simulink model "mcb_pmsm_foc_dual_host_model"  (R2024b)
settings: Solver=FixedStepDiscrete  StartTime=0.0  StopTime=inf  RelTol=1e-3  EnableMultiTasking=on
values from neighbouring files (symbols this model uses):
  dataType = 'single'    [mcb_pmsm_foc_dual_f28379d_datascript.m]    (also in mcb_pmsm_foc_sensorless_dyno_f28379d_datascript.m)
  PU_System = mcb_SetPUSystem(pmsm,inverter)    [mcb_pmsm_foc_dual_f28379d_datascript.m]
  Ts = T_pwm    (= 5e-05)    [mcb_pmsm_foc_dual_f28379d_datascript.m]    (also in mcb_pmsm_foc_sensorless_dyno_f28379d_datascript.m)
libraries: instrumentseriallib x4, simulink x3, demo_controls x1
settings Model: Creator=The MathWorks, Inc.  LastModifiedBy=36961
settings SolverCC: AlgebraicLoopSolver=TrustRegion  MaxZcPerStep=1
settings DataIOCC: LimitDataPoints=on  SaveFormat=Array  ReturnWorkspaceOutputs=off
settings OptimizationCC: LifeSpan=1  EfficientTunableParamExpr=on
settings DebuggingCC: UnderspecifiedInitializationDetection=Classic  MergeDetectMultiDrivingBlocksExec=none  SolverPrmCheckMsg=warning  ParameterPrecisionLossMsg=none  UnconnectedInputMsg=warning  UnconnectedOutputMsg=warning  UnconnectedLineMsg=warning  AllowSymbolicDim=off  PregeneratedLibrarySubsystemCodeDiagnostic=none  SFUnexpectedBacktrackingDiag=warning  SFNoUnconditionalDefaultTransitionDiag=warning  SFExecutionAtInitializationDiag=none  ArithmeticOperatorsInVariantConditions=warning
settings HardwareCC: ProdBitPerPointer=32  ProdLargestAtomicFloat=None  ProdIntDivRoundTo=Undefined  ProdEndianess=Unspecified  ProdWordSize=32  ProdHWDeviceType=32-bit Generic
settings ModelReferenceCC: EnableRefExpFcnMdlSchedulingChecks=on  PropagateSignalLabelsOutOfModel=off
settings SFSimCC: SimUseLocalCustomCode=off  MATLABDynamicMemAlloc=off
settings RTWCC: Description=Real-Time Workshop Embedded Coder  SystemTargetFile=ert.tlc  TemplateMakefile=ert_default_tmf  GenerateReport=on  RTWUseLocalCustomCode=off  IncludeHyperlinkInReport=on  LaunchReport=on  GenerateTraceInfo=on  GenerateTraceReport=on  GenerateTraceReportSl=on  GenerateTraceReportSf=on  GenerateTraceReportEml=on  GPUComputeCapability=3.5  DLArmComputeVersion=19.05
settings CodeAppCC: IgnoreCustomStorageClasses=off  StateflowObjectComments=on  InternalIdentifier=Classic
settings ERTTargetCC: MultiwordLength=2048  GenerateSampleERTMain=on  InlinedParameterPlacement=Hierarchical  ERTCustomFileTemplate=example_file_process.tlc  ConvertIfToSwitch=off  SuppressUnreachableDefaultCases=off  DynamicArrayContainerType=coder::array
settings ConfigComp: CovMetricSettings=dw  CovSaveCumulativeToWorkspaceVar=on  CovSaveSingleToWorkspaceVar=on  CovExternalEMLEnable=off  CovSFcnEnable=off

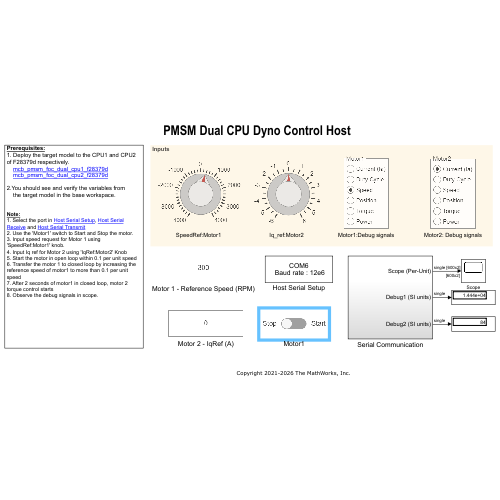
[thumbnail: Simulink's stored preview of the top-level diagram]
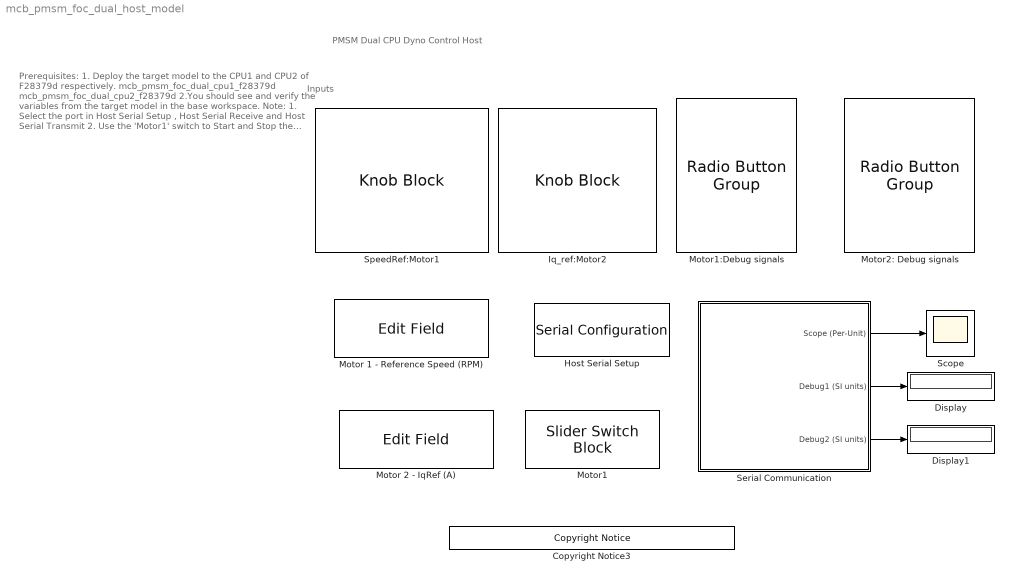
== system mcb_pmsm_foc_dual_host_model ==
  note: PMSM Dual CPU Dyno Control Host
  note: Prerequisites:
      | 1. Deploy the target model to the CPU1 and CPU2 of F28379d respectively.
      | mcb_pmsm_foc_dual_cpu1_f28379d
      | mcb_pmsm_foc_dual_cpu2_f28379d
      |
      | 2.You should see and verify the variables from
      | the target model in the base workspace.
      |
      | Note:
      | 1. Select the port in Host Serial Setup , Host Serial Receive and Host Serial Transmit
      | 2. Use the 'Motor1' switch to Start and Stop the motor.
      | 3. Input speed request for Motor 1 using 'SpeedRef:Motor1' knob.
      | 4. Input Iq ref for Motor 2 using 'IqRef:Motor2' Knob
      | 5. Start the motor in open loop within 0.1 per unit speed
      | 6. Transfer the motor 1 to closed loop by increasing the reference speed of motor1 to more than 0.1 per unit speed
      | 7. After 2 seconds of motor1 in closed loop, motor 2 torque control starts
      | 8. Observe the debug signals in scope.
  note: Inputs
  Copyright Notice3 : demo_controls/Copyright Notice  year=2021  prod=tic2000
  Display : Display
  Display1 : Display
  Host Serial Setup : instrumentseriallib/Serial Configuration  Priority=-99  PortSel=COM6  Port=COM6  ComPort=COM6  BaudRate=12e6  DataBits=8  Parity=none  StopBits=1  ByteOrder=little-endian  FlowControl=none  Timeout=2  SimulateUsing=Interpreted execution  BlockInModel=on  aMode=5
  Iq_ref:Motor2 : KnobBlock  LabelPosition=Hide  ScaleMin=-6  ScaleMax=6
  Motor 1 - Reference Speed (RPM) : EditField  LabelPosition=Hide  ShowInitialText=on  Alignment=Center
  Motor 2 - IqRef (A) : EditField  LabelPosition=Hide  ShowInitialText=on  Alignment=Center
  Motor1 : SliderSwitchBlock  LabelPosition=Hide
      settings: Values={{'Stop', 'Start'}, [0 1]}
  Motor1:Debug signals : RadioButtonGroup  LabelPosition=Hide  SelectedLabel=Speed  ButtonGroupName=Motor1
      settings: Values={{'Current (Ia)', 'Duty Cycle', 'Speed', 'Position', 'Torque', 'Power'}, [0 1 2 3 4 5]}
  Motor2: Debug signals : RadioButtonGroup  LabelPosition=Hide  SelectedLabel=Current (Ia)  ButtonGroupName=Motor2
      settings: Values={{'Current (Ia)', 'Duty Cycle', 'Speed', 'Position', 'Torque', 'Power'}, [0 1 2 3 4 5]}
  Scope : Scope
  Serial Communication : Subsystem
  SpeedRef:Motor1 : KnobBlock  LabelPosition=Hide  ScaleMin=-4000  ScaleMax=4000
  wires:
  Serial Communication/2(Debug1 (SI units)) -> Display/1
  Serial Communication/3(Debug2 (SI units)) -> Display1/1
  Serial Communication/1(Scope (Per-Unit)) -> Scope/1

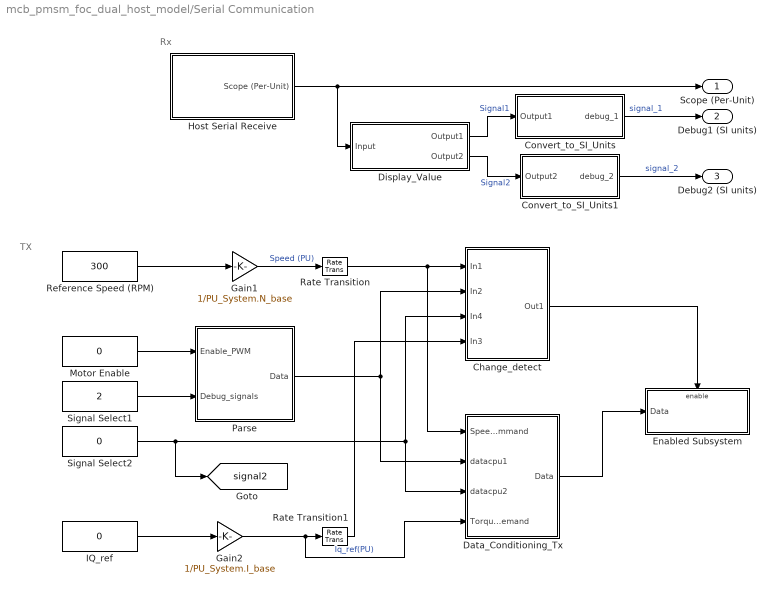
== system mcb_pmsm_foc_dual_host_model/Serial Communication ==
  note: TX
  note: Rx
  Change_detect : Subsystem
  Convert_to_SI_Units : Subsystem
  Convert_to_SI_Units1 : Subsystem
  Data_Conditioning_Tx : Subsystem  Variant=on
  Display_Value : MATLAB Function  TreatAsAtomicUnit=on
  Enabled Subsystem : Subsystem  TreatAsAtomicUnit=on
  Gain1 : Gain  Gain=1/PU_System.N_base  RndMeth=Simplest  OutDataTypeStr=Inherit: Same as input
  Gain2 : Gain  Gain=1/PU_System.I_base  RndMeth=Simplest  OutDataTypeStr=Inherit: Same as input
  Host Serial Receive : Subsystem  Variant=on
  IQ_ref : Constant  Value=0  VectorParams1D=off  OutDataTypeStr=single  SampleTime=0.03
  Motor Enable : Constant  Value=0  VectorParams1D=off  OutDataTypeStr=uint16  SampleTime=0.03
  Parse : Subsystem
  Rate Transition : RateTransition  OutPortSampleTime=0.03
  Rate Transition1 : RateTransition  OutPortSampleTime=0.03
  Reference Speed (RPM) : Constant  Value=300  VectorParams1D=off  OutDataTypeStr=single  SampleTime=0.03
  Signal Select1 : Constant  Value=2  OutDataTypeStr=uint16  SampleTime=0.03
  Signal Select2 : Constant  Value=0  OutDataTypeStr=uint16  SampleTime=0.03
  Scope (Per-Unit) : Outport
  Debug1 (SI units) : Outport  Port=2
  Debug2 (SI units) : Outport  Port=3
  tag scope: signal2=global
  wires:
  Reference Speed (RPM)/1 -> Gain1/1
  Gain2/1 -> Data_Conditioning_Tx/4(TorqueDemand), Rate Transition1/1  "Iq_ref(PU)"
  Parse/1(Data) -> Change_detect/2(In2), Data_Conditioning_Tx/2(datacpu1)
  Change_detect/1(Out1) -> Enabled Subsystem/Enable
  Data_Conditioning_Tx/1(Data) -> Enabled Subsystem/1(Data)
  Signal Select2/1 -> [signal2], Data_Conditioning_Tx/3(datacpu2), Change_detect/3(In4)
  Rate Transition1/1 -> Change_detect/4(In3)
  Motor Enable/1 -> Parse/1(Enable_PWM)
  IQ_ref/1 -> Gain2/1
  Gain1/1 -> Rate Transition/1  "Speed (PU)"
  Rate Transition/1 -> Data_Conditioning_Tx/1(SpeedCommand), Change_detect/1(In1)
  Signal Select1/1 -> Parse/2(Debug_signals)
  Display_Value/2(Output2) -> Convert_to_SI_Units1/1(Output2)  "Signal2"
  Display_Value/1(Output1) -> Convert_to_SI_Units/1(Output1)  "Signal1"
  Convert_to_SI_Units1/1(debug_2) -> Debug2 (SI units)/1  "signal_2"
  Host Serial Receive/1(Scope (Per-Unit)) -> Display_Value/1(Input), Scope (Per-Unit)/1
  Convert_to_SI_Units/1(debug_1) -> Debug1 (SI units)/1  "signal_1"

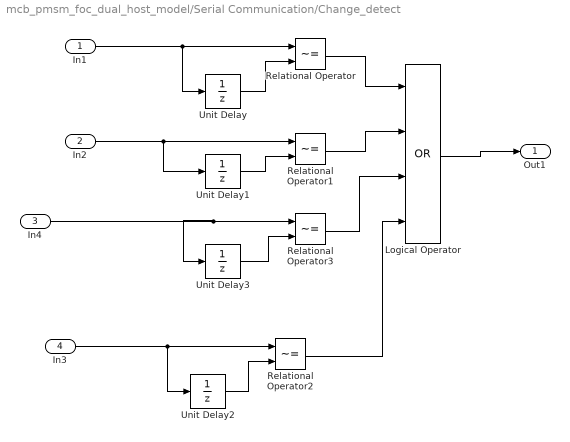
== system mcb_pmsm_foc_dual_host_model/Serial Communication/Change_detect ==
  In1 : Inport
  In2 : Inport  Port=2
  In4 : Inport  Port=3
  In3 : Inport  Port=4
  Logical Operator : Logic  Operator=OR  Inputs=4  AllPortsSameDT=off  OutDataTypeStr=boolean
  Relational Operator{,1..3} (4 alike) : RelationalOperator  Operator=~=  OutDataTypeStr=boolean  InputSameDT=off
  Unit Delay : UnitDelay  InitialCondition=0.5  SampleTime=-1  HasFrameUpgradeWarning=on
  Unit Delay1 : UnitDelay  SampleTime=-1  HasFrameUpgradeWarning=on
  Unit Delay2 : UnitDelay  InitialCondition=0.5  SampleTime=-1  HasFrameUpgradeWarning=on
  Unit Delay3 : UnitDelay  SampleTime=-1  HasFrameUpgradeWarning=on
  Out1 : Outport  VectorParamsAs1DForOutWhenUnconnected=off
  wires:
  In2/1 -> Relational Operator1/1, Unit Delay1/1
  Relational Operator1/1 -> Logical Operator/2
  Unit Delay1/1 -> Relational Operator1/2
  Unit Delay/1 -> Relational Operator/2
  In1/1 -> Unit Delay/1, Relational Operator/1
  Relational Operator/1 -> Logical Operator/1
  Logical Operator/1 -> Out1/1
  Relational Operator2/1 -> Logical Operator/4
  Unit Delay2/1 -> Relational Operator2/2
  In3/1 -> Unit Delay2/1, Relational Operator2/1
  In4/1 -> Relational Operator3/1, Unit Delay3/1
  Unit Delay3/1 -> Relational Operator3/2
  Relational Operator3/1 -> Logical Operator/3

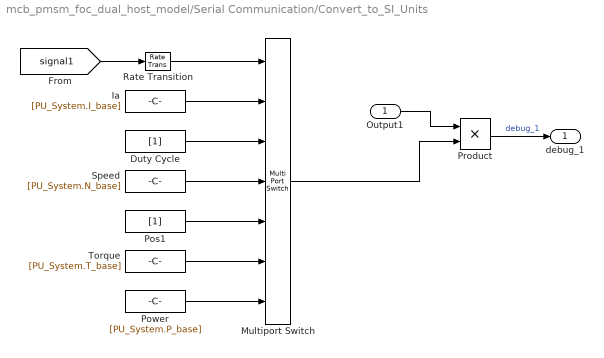
== system mcb_pmsm_foc_dual_host_model/Serial Communication/Convert_to_SI_Units ==
  Output1 : Inport
  Duty Cycle : Constant  Value=[1]  OutDataTypeStr=uint16  SampleTime=-1
  Ia : Constant  Value=[PU_System.I_base]  OutDataTypeStr=uint16  SampleTime=-1
  Multiport Switch : MultiPortSwitch  DataPortOrder=Zero-based contiguous  Inputs=6  DiagnosticForDefault=Warning  zeroidx=on  OutDataTypeStr=uint16  RndMeth=Simplest  SaturateOnIntegerOverflow=off  InputSameDT=off
  Pos1 : Constant  Value=[1]  OutDataTypeStr=uint16  SampleTime=-1
  Power : Constant  Value=[PU_System.P_base]  OutDataTypeStr=uint16  SampleTime=-1
  Product : Product
  Rate Transition : RateTransition  Deterministic=off
  Speed : Constant  Value=[PU_System.N_base]  OutDataTypeStr=uint16  SampleTime=-1
  Torque : Constant  Value=[PU_System.T_base]  OutDataTypeStr=uint16  SampleTime=-1
  debug_1 : Outport
  wires:
  Product/1 -> debug_1/1  "debug_1"
  [signal1] -> Rate Transition/1
  Output1/1 -> Product/1
  Rate Transition/1 -> Multiport Switch/1
  Pos1/1 -> Multiport Switch/5
  Speed/1 -> Multiport Switch/4
  Duty Cycle/1 -> Multiport Switch/3
  Ia/1 -> Multiport Switch/2
  Multiport Switch/1 -> Product/2
  Torque/1 -> Multiport Switch/6
  Power/1 -> Multiport Switch/7

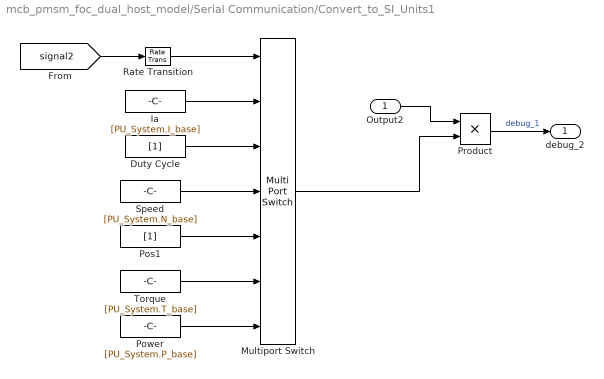
== system mcb_pmsm_foc_dual_host_model/Serial Communication/Convert_to_SI_Units1 ==
  Output2 : Inport
  Duty Cycle : Constant  Value=[1]  OutDataTypeStr=uint16  SampleTime=-1
  Ia : Constant  Value=[PU_System.I_base]  OutDataTypeStr=uint16  SampleTime=-1
  Multiport Switch : MultiPortSwitch  DataPortOrder=Zero-based contiguous  Inputs=6  DiagnosticForDefault=Warning  zeroidx=on  OutDataTypeStr=uint16  RndMeth=Simplest  SaturateOnIntegerOverflow=off  InputSameDT=off
  Pos1 : Constant  Value=[1]  OutDataTypeStr=uint16  SampleTime=-1
  Power : Constant  Value=[PU_System.P_base]  OutDataTypeStr=uint16  SampleTime=-1
  Product : Product
  Rate Transition : RateTransition  Deterministic=off
  Speed : Constant  Value=[PU_System.N_base]  OutDataTypeStr=uint16  SampleTime=-1
  Torque : Constant  Value=[PU_System.T_base]  OutDataTypeStr=uint16  SampleTime=-1
  debug_2 : Outport
  wires:
  Multiport Switch/1 -> Product/2
  Ia/1 -> Multiport Switch/2
  Duty Cycle/1 -> Multiport Switch/3
  Speed/1 -> Multiport Switch/4
  Pos1/1 -> Multiport Switch/5
  Rate Transition/1 -> Multiport Switch/1
  Output2/1 -> Product/1
  [signal2] -> Rate Transition/1
  Product/1 -> debug_2/1  "debug_1"
  Power/1 -> Multiport Switch/7
  Torque/1 -> Multiport Switch/6

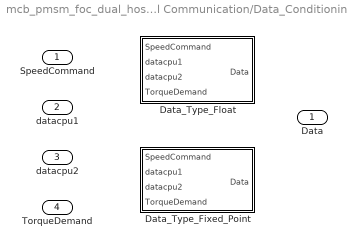
== system mcb_pmsm_foc_dual_host_model/Serial Communication/Data_Conditioning_Tx ==
  SpeedCommand : Inport
  datacpu1 : Inport  Port=2
  datacpu2 : Inport  Port=3
  TorqueDemand : Inport  Port=4
  Data_Type_Fixed_Point : Subsystem  VariantControl=~isequal(dataType, 'single')
  Data_Type_Float : Subsystem  VariantControl=isequal(dataType, 'single')
  Data : Outport

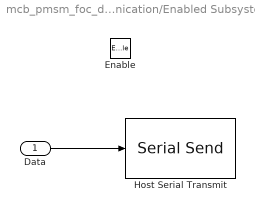
== system mcb_pmsm_foc_dual_host_model/Serial Communication/Enabled Subsystem ==
  Data : Inport
  Enable : EnablePort
  Host Serial Transmit : instrumentseriallib/Serial Send  PortSel=COM6  Port=COM6  ComPort=COM6  Header=[]  Terminator=<none>  CustomTerminator=[]  EnableBlockingMode=off  SimulateUsing=Interpreted execution  BlockInModel=on  aMode=5
  wires:
  Data/1 -> Host Serial Transmit/1

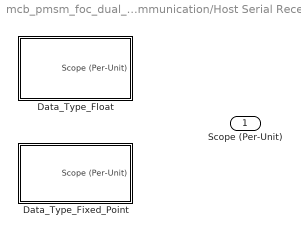
== system mcb_pmsm_foc_dual_host_model/Serial Communication/Host Serial Receive ==
  Data_Type_Fixed_Point : Subsystem  VariantControl=~isequal(dataType, 'single')
  Data_Type_Float : Subsystem  VariantControl=isequal(dataType, 'single')
  Scope (Per-Unit) : Outport

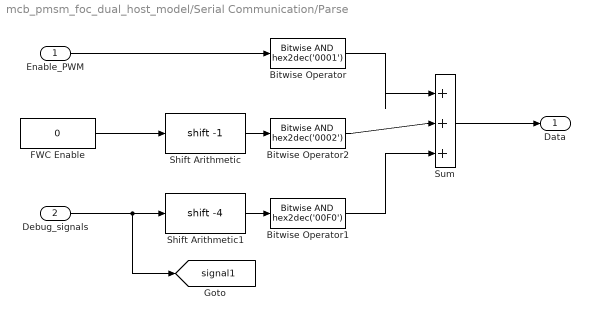
== system mcb_pmsm_foc_dual_host_model/Serial Communication/Parse ==
  Enable_PWM : Inport
  Debug_signals : Inport  Port=2
  Bitwise Operator : simulink/Logic and Bit Operations/Bitwise Operator  logicop=AND  UseBitMask=on  BitMask=hex2dec('0001')  BitMaskRealWorld=Stored Integer
  Bitwise Operator1 : simulink/Logic and Bit Operations/Bitwise Operator  logicop=AND  UseBitMask=on  BitMask=hex2dec('00F0')  BitMaskRealWorld=Stored Integer
  Bitwise Operator2 : simulink/Logic and Bit Operations/Bitwise Operator  logicop=AND  UseBitMask=on  BitMask=hex2dec('0002')  BitMaskRealWorld=Stored Integer
  FWC Enable : Constant  Value=0  VectorParams1D=off  OutDataTypeStr=uint16  SampleTime=0.03
  Shift Arithmetic : ArithShift  BitShiftNumber=-1
  Shift Arithmetic1 : ArithShift  BitShiftNumber=-4
  Sum : Sum  Inputs=|+++
  Data : Outport
  tag scope: signal1=global
  wires:
  Bitwise Operator/1 -> Sum/1
  Debug_signals/1 -> [signal1], Shift Arithmetic1/1
  Sum/1 -> Data/1
  Shift Arithmetic1/1 -> Bitwise Operator1/1
  Shift Arithmetic/1 -> Bitwise Operator2/1
  Bitwise Operator1/1 -> Sum/3
  FWC Enable/1 -> Shift Arithmetic/1
  Bitwise Operator2/1 -> Sum/2
  Enable_PWM/1 -> Bitwise Operator/1

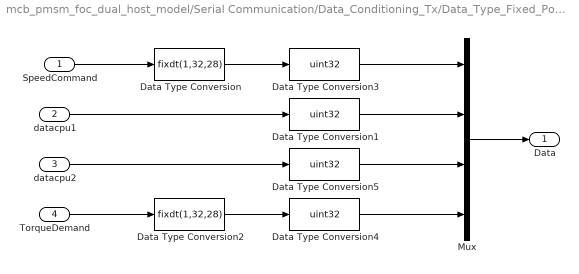
== system mcb_pmsm_foc_dual_host_model/Serial Communication/Data_Conditioning_Tx/Data_Type_Fixed_Point ==
  SpeedCommand : Inport
  datacpu1 : Inport  Port=2
  datacpu2 : Inport  Port=3
  TorqueDemand : Inport  Port=4
  Data Type Conversion : DataTypeConversion  OutDataTypeStr=fixdt(1,32,28)  RndMeth=Simplest  SaturateOnIntegerOverflow=off
  Data Type Conversion1 : DataTypeConversion  OutDataTypeStr=uint32  RndMeth=Simplest  SaturateOnIntegerOverflow=off
  Data Type Conversion2 : DataTypeConversion  OutDataTypeStr=fixdt(1,32,28)  RndMeth=Simplest  SaturateOnIntegerOverflow=off
  Data Type Conversion3 : DataTypeConversion  OutDataTypeStr=uint32  ConvertRealWorld=Stored Integer (SI)  RndMeth=Simplest  SaturateOnIntegerOverflow=off
  Data Type Conversion4 : DataTypeConversion  OutDataTypeStr=uint32  ConvertRealWorld=Stored Integer (SI)  RndMeth=Simplest  SaturateOnIntegerOverflow=off
  Data Type Conversion5 : DataTypeConversion  OutDataTypeStr=uint32  RndMeth=Simplest  SaturateOnIntegerOverflow=off
  Mux : Mux
  Data : Outport
  wires:
  SpeedCommand/1 -> Data Type Conversion/1
  Data Type Conversion3/1 -> Mux/1
  Data Type Conversion/1 -> Data Type Conversion3/1
  datacpu1/1 -> Data Type Conversion1/1
  Data Type Conversion1/1 -> Mux/2
  Mux/1 -> Data/1
  Data Type Conversion2/1 -> Data Type Conversion4/1
  Data Type Conversion4/1 -> Mux/4
  Data Type Conversion5/1 -> Mux/3
  datacpu2/1 -> Data Type Conversion5/1
  TorqueDemand/1 -> Data Type Conversion2/1

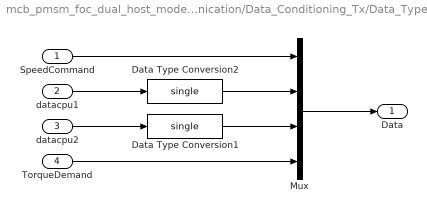
== system mcb_pmsm_foc_dual_host_model/Serial Communication/Data_Conditioning_Tx/Data_Type_Float ==
  SpeedCommand : Inport
  datacpu1 : Inport  Port=2
  datacpu2 : Inport  Port=3
  TorqueDemand : Inport  Port=4
  Data Type Conversion1 : DataTypeConversion  OutDataTypeStr=single  RndMeth=Simplest  SaturateOnIntegerOverflow=off
  Data Type Conversion2 : DataTypeConversion  OutDataTypeStr=single  RndMeth=Simplest  SaturateOnIntegerOverflow=off
  Mux : Mux
  Data : Outport
  wires:
  SpeedCommand/1 -> Mux/1
  Mux/1 -> Data/1
  datacpu1/1 -> Data Type Conversion2/1
  Data Type Conversion2/1 -> Mux/2
  datacpu2/1 -> Data Type Conversion1/1
  Data Type Conversion1/1 -> Mux/3
  TorqueDemand/1 -> Mux/4

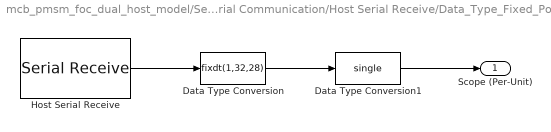
== system mcb_pmsm_foc_dual_host_model/Serial Communication/Host Serial Receive/Data_Type_Fixed_Point ==
  Data Type Conversion : DataTypeConversion  OutDataTypeStr=fixdt(1,32,28)  ConvertRealWorld=Stored Integer (SI)  RndMeth=Simplest  SaturateOnIntegerOverflow=off
  Data Type Conversion1 : DataTypeConversion  OutDataTypeStr=single  RndMeth=Simplest  SaturateOnIntegerOverflow=off
  Host Serial Receive : instrumentseriallib/Serial Receive  PortSel=<Select a port...>  Port=<Select a port...>  ComPort=<Select a port...>  DataType=uint32  SaveDataType=uint8  ToggleHeader=on  Header='SSSS'  ToggleDataSize=on  DataSize=[600 2]  ToggleTerminator=on  Terminator=Custom terminator  CustomTerminator='EEEE'  InputFormat=Row major  EnableBlockingMode=on  ActionDataUnavailable=Output custom value  ActionWhenDataUnavailable=Output custom value  CustomValue=4  SampleTime=600*Ts  SimulateUsing=Interpreted execution  BlockInModel=on  aMode=5
  Scope (Per-Unit) : Outport
  wires:
  Data Type Conversion/1 -> Data Type Conversion1/1
  Host Serial Receive/1 -> Data Type Conversion/1
  Data Type Conversion1/1 -> Scope (Per-Unit)/1

== system mcb_pmsm_foc_dual_host_model/Serial Communication/Host Serial Receive/Data_Type_Float ==
  Host Serial Receive : instrumentseriallib/Serial Receive  PortSel=COM6  Port=COM6  ComPort=COM6  DataType=single  SaveDataType=uint8  ToggleHeader=on  Header='SSSS'  ToggleDataSize=on  DataSize=[600 2]  ToggleTerminator=on  Terminator=Custom terminator  CustomTerminator='EEEE'  InputFormat=Row major  EnableBlockingMode=on  ActionDataUnavailable=Output custom value  ActionWhenDataUnavailable=Output custom value  CustomValue=4  SampleTime=600*Ts  SimulateUsing=Interpreted execution  BlockInModel=on  aMode=5
  Scope (Per-Unit) : Outport
  wires:
  Host Serial Receive/1 -> Scope (Per-Unit)/1

== matlab function mcb_pmsm_foc_dual_host_model/Serial Communication/Display_Value ==
  data: Output1 output; Input input; Output2 output
function [Output1, Output2] = unBuf (Input)
%% ************************************************************************
% Unbuffer function
% Outputs first received serial data from buffer for both signals

% Copyright 2020 The MathWorks, Inc.

selSignal= Input(:, 1);
Output1 = selSignal(1,1);
selSignal = Input(:, 2);
Output2 = selSignal(1,1);
end
